simulink model "debug_ev3"  (R2023a)
settings: Solver=FixedStepAuto  StartTime=0.0  StopTime=13  RelTol=1e-3  EnableMultiTasking=on
undefined symbols (not defined in the file): R_1_front, R_1_side, Ts
libraries: legoev3lib x11
settings Model: ExtModeTrigDuration=2  Creator=morit  LastModifiedBy=morit
settings SolverCC: PositivePriorityOrder=on
settings OptimizationCC: EnhancedBackFolding=on  PassReuseOutputArgsAs=Individual arguments  ZeroExternalMemoryAtStartup=off  ZeroInternalMemoryAtStartup=off  MaxStackSize=64  OptimizeBlockOrder=speed  DifferentSizesBufferReuse=on  OptimizationCustomize=off  EfficientTunableParamExpr=on
settings DebuggingCC: ParameterTunabilityLossMsg=error
settings HardwareCC: ProdBitPerPointer=32  ProdBitPerSizeT=32  ProdBitPerPtrDiffT=32  ProdLargestAtomicInteger=Long  ProdWordSize=32  ProdHWDeviceType=ARM Compatible->ARM 9
settings SFSimCC: MATLABDynamicMemAlloc=off
settings RTWCC: Description=Embedded Coder  SystemTargetFile=ert.tlc  HardwareBoard=LEGO MINDSTORMS EV3  TLCOptions="-aInlineSetEventsForThisBaseRateFcn=TLC_FALSE -aSuppressMultiTaskScheduler=TLC_FALSE  -aRateBasedStepFcn=0"  TemplateMakefile=ert_default_tmf  Toolchain=Sourcery G++ Lite v2009q3
settings CodeAppCC: ForceParamTrailComments=on  IgnoreCustomStorageClasses=off  OperatorAnnotations=on  SimulinkDataObjDesc=on  SFDataObjDesc=on  InsertBlockDesc=on
settings ERTTargetCC: SupportContinuousTime=on  SupportVariableSizeSignals=on  ExtModeTransport=2  ExtModeStaticAlloc=on  ExtModeMexFile=ext_xcp  ExtModeIntrfLevel=Level2 - Open

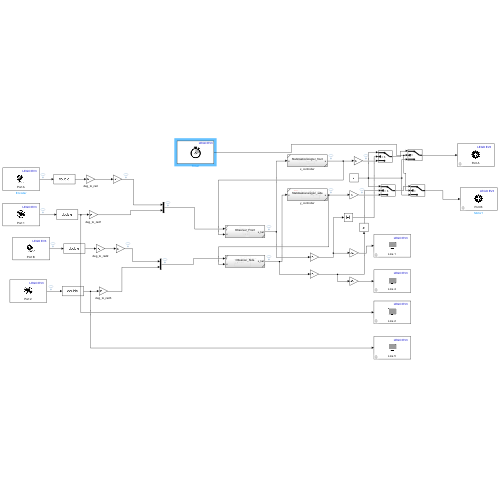
[thumbnail: Simulink's stored preview of the top-level diagram]
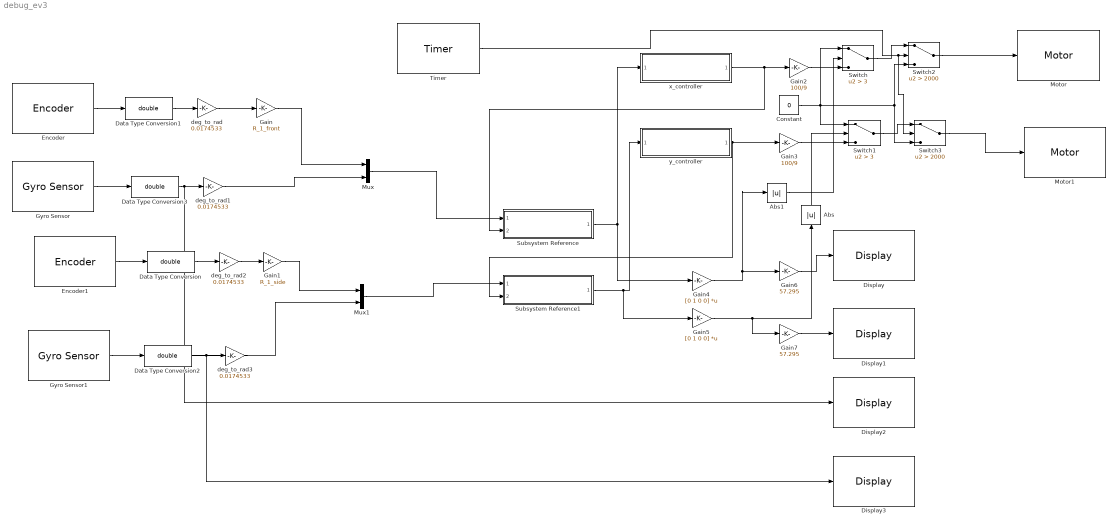
== system debug_ev3 ==
  Abs : Abs  SaturateOnIntegerOverflow=off
  Abs1 : Abs  SaturateOnIntegerOverflow=off
  Constant : Constant  Value=0
  Data Type Conversion{,1..3} (4 alike) : DataTypeConversion  OutDataTypeStr=double  SaturateOnIntegerOverflow=off  RndMeth=Floor
  Display : legoev3lib/Display  slcdLine=1  slcdFormat=Decimal
  Display1 : legoev3lib/Display  slcdLine=4  slcdFormat=Decimal
  Display2 : legoev3lib/Display  slcdLine=2  slcdFormat=Decimal
  Display3 : legoev3lib/Display  slcdLine=5  slcdFormat=Decimal
  Encoder : legoev3lib/Encoder  portNumber=A  opMode=Reset at each sample time  sampleTime=Ts
  Encoder1 : legoev3lib/Encoder  portNumber=B  opMode=Reset at each sample time  sampleTime=Ts
  Gain : Gain  Gain=R_1_front
  Gain1 : Gain  Gain=R_1_side
  Gain2 : Gain  Gain=100/9
  Gain3 : Gain  Gain=100/9
  Gain4 : Gain  Gain=[0 1 0 0]  Multiplication=Matrix(K*u)
  Gain5 : Gain  Gain=[0 1 0 0]  Multiplication=Matrix(K*u)
  Gain6 : Gain  Gain=57.295
  Gain7 : Gain  Gain=57.295
  Gyro Sensor : legoev3lib/Gyro Sensor  portNumber=1  sampleTime=Ts
  Gyro Sensor1 : legoev3lib/Gyro Sensor  portNumber=2  sampleTime=Ts
  Motor : legoev3lib/Motor  sportNumber=A  sstopAction=Brake
  Motor1 : legoev3lib/Motor  sportNumber=B  sstopAction=Brake
  Mux : Mux  Inputs=2
  Mux1 : Mux  Inputs=2
  Subsystem Reference : Subsystem  ReferencedSubsystem=Observer_Front
  Subsystem Reference1 : Subsystem  ReferencedSubsystem=Observer_Side
  Switch : Switch  Criteria=u2 > Threshold  Threshold=3  SaturateOnIntegerOverflow=off  InputSameDT=off
  Switch1 : Switch  Criteria=u2 > Threshold  Threshold=3  SaturateOnIntegerOverflow=off  InputSameDT=off
  Switch2 : Switch  Criteria=u2 > Threshold  Threshold=2000  SaturateOnIntegerOverflow=off  InputSameDT=off
  Switch3 : Switch  Criteria=u2 > Threshold  Threshold=2000  SaturateOnIntegerOverflow=off  InputSameDT=off
  Timer : legoev3lib/Timer  SampleTime=Ts
  deg_to_rad{,1..3} (4 alike) : Gain  Gain=0.0174533
  x_controller : Subsystem  ReferencedSubsystem=Stabilisationsregler_front
  y_controller : Subsystem  ReferencedSubsystem=Stabilisationsregler_side
  wires:
  Mux/1 -> Subsystem Reference/1
  Gain/1 -> Mux/1
  Encoder1/1 -> Data Type Conversion/1
  Gyro Sensor1/1 -> Data Type Conversion2/1
  Subsystem Reference1/1 -> Gain5/1, y_controller/1
  y_controller/1 -> Subsystem Reference1/2, Gain3/1
  Mux1/1 -> Subsystem Reference1/1
  Gain1/1 -> Mux1/1
  Gyro Sensor/1 -> Data Type Conversion3/1
  Encoder/1 -> Data Type Conversion1/1
  Subsystem Reference/1 -> x_controller/1, Gain4/1
  x_controller/1 -> Subsystem Reference/2, Gain2/1
  Data Type Conversion/1 -> deg_to_rad2/1
  Data Type Conversion1/1 -> deg_to_rad/1
  Data Type Conversion2/1 -> Display3/1, deg_to_rad3/1
  Data Type Conversion3/1 -> Display2/1, deg_to_rad1/1
  deg_to_rad/1 -> Gain/1
  deg_to_rad1/1 -> Mux/2
  deg_to_rad2/1 -> Gain1/1
  deg_to_rad3/1 -> Mux1/2
  Gain5/1 -> Abs/1, Gain7/1
  Gain4/1 -> Gain6/1, Abs1/1
  Gain2/1 -> Switch/3
  Gain3/1 -> Switch1/3
  Constant/1 -> Switch3/3, Switch2/3, Switch/1, Switch1/1
  Gain6/1 -> Display/1
  Gain7/1 -> Display1/1
  Abs/1 -> Switch1/2
  Abs1/1 -> Switch/2
  Switch/1 -> Switch2/1
  Switch2/1 -> Motor/1
  Switch3/1 -> Motor1/1
  Switch1/1 -> Switch3/1
  Timer/1 -> Switch3/2, Switch2/2
